simulink model "EulerPIDJoint_Tmp"  (Simulink 7.6)
settings: Solver=ode45  StartTime=0.0  StopTime=8  RelTol=1e-3
InitFcn:
  | eval('Config')
values from neighbouring files (symbols this model uses):
  a2 = 0    [Config.m]    (also in CtrPlatformCfg.m)
  a3 = 0    [Config.m]    (also in CtrPlatformCfg.m)
  a4 = 0    [Config.m]    (also in CtrPlatformCfg.m)
  a5 = 90    [Config.m]    (also in CtrPlatformCfg.m)
  a6 = 0    [Config.m]    (also in CtrPlatformCfg.m)
  Cen_EU = Cen    [DynEulerTest.m]
  DH_EU = [266     300     0       0       1016     0      174 ... (first row only)    [DynEulerTest.m]
  freq = tvel/radius    (= 1)    [Config.m]    (also in CtrPlatformCfg.m)
  Ft_EU = [0;0;0;0;0;0]    [DynEulerTest.m]
  Gravity = 9.8    [Config.m]    (also in CtrPlatformCfg.m)
  Ie_EU = [Ie1;Ie2;Ie3;Ie4;Ie5;Ie6]    [DynEulerTest.m]
  in1 = [5.2954 -0.2565 -0.6366;-0.2565 4.7000 0.2830;-0.6366 0.2829 5.8635]    [Config.m]    (also in CtrPlatformCfg.m; DynEulerTest.m; EfDynCAD.m = [0.54  -0.01 0.23)
  in2 = [5.8840 0.0072 0.0135;0.0072 6.0178 -0.1907;0.0135 -0.1907 0.3374]    [Config.m]    (also in CtrPlatformCfg.m; DynEulerTest.m; EfDynCAD.m = (R_x*R_z)*in2*(R_x*R_z)')
  in3 = [1.8201 -0.2274 -0.3112;-0.2274 2.2537 -0.1441;-0.3112 -0.1441 1.9485]    [Config.m]    (also in CtrPlatformCfg.m; DynEulerTest.m; EfDynCAD.m = (R_x*R_z)*in3*(R_x*R_z)')
  in4 = [0.0607 -0.0922 0;-0.0922 1.4493 0;0 0 1.4620]    [Config.m]    (also in CtrPlatformCfg.m; DynEulerTest.m = [0.0607 -0.0922 0;-0.0922 1.4493 0;0 0,1.4620]; EfDynCAD.m = (R_y*Rz)*in4*(R_y*Rz)')
  in5 = [0.0191 0.0032 0;0.0032 0.0228 0;0 0 0.0291]    [Config.m]    (also in CtrPlatformCfg.m; DynEulerTest.m; EfDynCAD.m = (R_x*R_y)*in5*(R_x*R_y)')
  in6 = [0.0012 0 0;0 0.0007 0;0 0 0.0007]    [Config.m]    (also in CtrPlatformCfg.m; DynEulerTest.m; EfDynCAD.m = (R_y*Rz)*in6*(R_y*Rz)')
  init_Endx = gd_init(1,4)    [Config.m]    (also in CtrPlatformCfg.m)
  init_Endy = gd_init(2,4)    [Config.m]    (also in CtrPlatformCfg.m)
  init_Endz = gd_init(3,4)    [Config.m]    (also in CtrPlatformCfg.m)
  init_Rot = gd_init(1:3,1:3)    [Config.m]    (also in CtrPlatformCfg.m)
  L = [l1 l2 l3 l4 l5 l6 l7 l8 l9]    [Config.m]    (also in CtrPlatformCfg.m)
  ma1 = 170.31    [Config.m]    (also in CtrPlatformCfg.m; DynEulerTest.m; EfDynCAD.m = 77.75)
  ma2 = 63.74    [Config.m]    (also in CtrPlatformCfg.m; DynEulerTest.m; EfDynCAD.m = 32.31)
  ma3 = 98.98    [Config.m]    (also in CtrPlatformCfg.m; DynEulerTest.m; EfDynCAD.m = 18.61)
  ma4 = 24.46    [Config.m]    (also in CtrPlatformCfg.m; DynEulerTest.m; EfDynCAD.m = 15.65)
  ma5 = 5.24    [Config.m]    (also in CtrPlatformCfg.m; DynEulerTest.m; EfDynCAD.m = 3.32)
  ma6 = 0.6    [Config.m]    (also in CtrPlatformCfg.m; DynEulerTest.m; EfDynCAD.m)
  Ma_EU = Ma    [DynEulerTest.m]
  tvel = 120    [Config.m]    (also in CtrPlatformCfg.m)
undefined symbols (not defined in the file or in its folder): a1
libraries: mblibv1 x41, simulink x4
(part 3 of 4)

== system EulerPIDJoint_Tmp/Display/GeneralVelDisplay/Jnt6 ==
  Enc : Inport
  Ref : Inport  Port=2
  Demux1 : Demux  Outputs=2
  Demux3 : Demux  Outputs=6
  Display : Subsystem
  Mux : Mux  Inputs=3
  Mux1 : Mux  Inputs=3
  Mux2 : Mux  Inputs=2
  Mux3 : Mux  Inputs=2
  Sign{1,3..4,6} (4 alike) : Gain
  Sign2 : Gain  Gain=-1
  Sign5 : Gain  Gain=-1
  wires:
  Mux3/1 -> Display/2(Ref_GeneralVel6)
  Mux2/1 -> Display/1(GeneralVel6)
  Sign5/1 -> Mux1/2
  Sign2/1 -> Mux/2
  Demux3/6 -> Sign6/1
  Demux3/5 -> Sign5/1
  Demux3/4 -> Sign4/1
  Demux3/3 -> Sign3/1
  Demux3/2 -> Sign2/1
  Demux3/1 -> Sign1/1
  Mux1/1 -> Mux3/2
  Mux/1 -> Mux3/1
  Ref/1 -> Demux3/1
  Enc/1 -> Demux1/1
  Sign1/1 -> Mux/3
  Sign3/1 -> Mux/1
  Sign6/1 -> Mux1/1
  Sign4/1 -> Mux1/3
  Demux1/1 -> Mux2/1
  Demux1/2 -> Mux2/2

== system EulerPIDJoint_Tmp/Display/JntVelAccDisplay/Joint1 ==
  JVA1 : Inport
  Ref_JVA1 : Inport  Port=2
  Acceleration : Scope  NumInputPorts=2
      settings: YMin=-5~-5  YMax=5~5  SaveName=ScopeData2
  Angle : Scope  NumInputPorts=2
      settings: TimeRange=10  YMin=-2.999999999999999e-017~-1  YMax=4e-017~1
  Demux : Demux  Outputs=3
  Demux1 : Demux  Outputs=3
  "Encoder " : ToWorkspace  VariableName=EncJVAJ1  SampleTime=-1  SaveFormat=Structure
  Err1 : Scope
      settings: SaveName=ScopeData6
  Err2 : Scope
      settings: SaveName=ScopeData7
  Err3 : Scope
      settings: SaveName=ScopeData8
  "Ref " : ToWorkspace  VariableName=RefJVAJ1  SampleTime=-1  SaveFormat=Structure
  Sum : Sum  Inputs=+|-
  Sum1 : Sum  Inputs=+|-
  Sum2 : Sum  Inputs=+|-
  "Velocity " : Scope  NumInputPorts=2
      settings: YMin=-5~-5  YMax=5~5
  wires:
  Ref_JVA1/1 -> "Ref "/1, Demux1/1
  JVA1/1 -> "Encoder "/1, Demux/1
  Sum2/1 -> Err3/1
  Sum1/1 -> Err2/1
  Sum/1 -> Err1/1
  Demux/1 -> Angle/1, Sum/1
  Demux1/1 -> Angle/2, Sum/2
  Demux/2 -> "Velocity "/1, Sum1/1
  Demux1/2 -> "Velocity "/2, Sum1/2
  Demux/3 -> Acceleration/1, Sum2/1
  Demux1/3 -> Acceleration/2, Sum2/2

== system EulerPIDJoint_Tmp/Display/JntVelAccDisplay/Joint2 ==
  JVA2 : Inport
  Ref_JVA2 : Inport  Port=2
  Acceleration : Scope  NumInputPorts=2
      settings: YMin=-5~-5  YMax=5~5  SaveName=ScopeData2
  Angle : Scope  NumInputPorts=2
      settings: TimeRange=10  YMin=-2.999999999999999e-017~-1  YMax=4e-017~1
  Demux : Demux  Outputs=3
  Demux1 : Demux  Outputs=3
  "Encoder " : ToWorkspace  VariableName=EncJVAJ2  SampleTime=-1  SaveFormat=Structure
  Err1 : Scope
      settings: SaveName=ScopeData6
  Err2 : Scope
      settings: SaveName=ScopeData7
  Err3 : Scope
      settings: SaveName=ScopeData8
  "Ref " : ToWorkspace  VariableName=RefJVAJ2  SampleTime=-1  SaveFormat=Structure
  Sum : Sum  Inputs=+|-
  Sum1 : Sum  Inputs=+|-
  Sum2 : Sum  Inputs=+|-
  "Velocity " : Scope  NumInputPorts=2
      settings: YMin=-5~-5  YMax=5~5
  wires:
  Demux1/3 -> Sum2/2, Acceleration/2
  Demux/3 -> Sum2/1, Acceleration/1
  Demux1/2 -> Sum1/2, "Velocity "/2
  Demux/2 -> Sum1/1, "Velocity "/1
  Demux1/1 -> Sum/2, Angle/2
  Demux/1 -> Sum/1, Angle/1
  Sum/1 -> Err1/1
  Sum1/1 -> Err2/1
  Sum2/1 -> Err3/1
  JVA2/1 -> Demux/1, "Encoder "/1
  Ref_JVA2/1 -> Demux1/1, "Ref "/1

== system EulerPIDJoint_Tmp/Display/JntVelAccDisplay/Joint3 ==
  JVA3 : Inport
  Ref_JVA3 : Inport  Port=2
  Acceleration : Scope  NumInputPorts=2
      settings: YMin=-5~-5  YMax=5~5  SaveName=ScopeData2
  Angle : Scope  NumInputPorts=2
      settings: TimeRange=10  YMin=-2.999999999999999e-017~-1  YMax=4e-017~1
  Demux : Demux  Outputs=3
  Demux1 : Demux  Outputs=3
  "Encoder " : ToWorkspace  VariableName=EncJVAJ3  SampleTime=-1  SaveFormat=Structure
  Err1 : Scope
      settings: SaveName=ScopeData6
  Err2 : Scope
      settings: SaveName=ScopeData7
  Err3 : Scope
      settings: SaveName=ScopeData8
  "Ref " : ToWorkspace  VariableName=RefJVAJ3  SampleTime=-1  SaveFormat=Structure
  Sum : Sum  Inputs=+|-
  Sum1 : Sum  Inputs=+|-
  Sum2 : Sum  Inputs=+|-
  "Velocity " : Scope  NumInputPorts=2
      settings: YMin=-5~-5  YMax=5~5
  wires:
  Ref_JVA3/1 -> "Ref "/1, Demux1/1
  JVA3/1 -> "Encoder "/1, Demux/1
  Sum2/1 -> Err3/1
  Sum1/1 -> Err2/1
  Sum/1 -> Err1/1
  Demux/1 -> Angle/1, Sum/1
  Demux1/1 -> Angle/2, Sum/2
  Demux/2 -> "Velocity "/1, Sum1/1
  Demux1/2 -> "Velocity "/2, Sum1/2
  Demux/3 -> Acceleration/1, Sum2/1
  Demux1/3 -> Acceleration/2, Sum2/2

== system EulerPIDJoint_Tmp/Display/JntVelAccDisplay/Joint4 ==
  JVA4 : Inport
  Ref_JVA4 : Inport  Port=2
  Acceleration : Scope  NumInputPorts=2
      settings: YMin=-5~-5  YMax=5~5  SaveName=ScopeData2
  Angle : Scope  NumInputPorts=2
      settings: TimeRange=10  YMin=-2.999999999999999e-017~-1  YMax=4e-017~1
  Demux : Demux  Outputs=3
  Demux1 : Demux  Outputs=3
  "Encoder " : ToWorkspace  VariableName=EncJVAJ4  SampleTime=-1  SaveFormat=Structure
  Err1 : Scope
      settings: SaveName=ScopeData6
  Err2 : Scope
      settings: SaveName=ScopeData7
  Err3 : Scope
      settings: SaveName=ScopeData8
  "Ref " : ToWorkspace  VariableName=RefJVAJ4  SampleTime=-1  SaveFormat=Structure
  Sum : Sum  Inputs=+|-
  Sum1 : Sum  Inputs=+|-
  Sum2 : Sum  Inputs=+|-
  "Velocity " : Scope  NumInputPorts=2
      settings: YMin=-5~-5  YMax=5~5
  wires:
  Demux1/3 -> Sum2/2, Acceleration/2
  Demux/3 -> Sum2/1, Acceleration/1
  Demux1/2 -> Sum1/2, "Velocity "/2
  Demux/2 -> Sum1/1, "Velocity "/1
  Demux1/1 -> Sum/2, Angle/2
  Demux/1 -> Sum/1, Angle/1
  Sum/1 -> Err1/1
  Sum1/1 -> Err2/1
  Sum2/1 -> Err3/1
  JVA4/1 -> Demux/1, "Encoder "/1
  Ref_JVA4/1 -> Demux1/1, "Ref "/1

== system EulerPIDJoint_Tmp/Display/JntVelAccDisplay/Joint5 ==
  JVA5 : Inport
  Ref_JVA5 : Inport  Port=2
  Acceleration : Scope  NumInputPorts=2
      settings: YMin=-5~-5  YMax=5~5  SaveName=ScopeData2
  Angle : Scope  NumInputPorts=2
      settings: TimeRange=10  YMin=-2.999999999999999e-017~-1  YMax=4e-017~1
  Demux : Demux  Outputs=3
  Demux1 : Demux  Outputs=3
  "Encoder " : ToWorkspace  VariableName=EncJVAJ5  SampleTime=-1  SaveFormat=Structure
  Err1 : Scope
      settings: SaveName=ScopeData6
  Err2 : Scope
      settings: SaveName=ScopeData7
  Err3 : Scope
      settings: SaveName=ScopeData8
  "Ref " : ToWorkspace  VariableName=RefJVAJ5  SampleTime=-1  SaveFormat=Structure
  Sum : Sum  Inputs=+|-
  Sum1 : Sum  Inputs=+|-
  Sum2 : Sum  Inputs=+|-
  "Velocity " : Scope  NumInputPorts=2
      settings: YMin=-5~-5  YMax=5~5
  wires:
  Ref_JVA5/1 -> "Ref "/1, Demux1/1
  JVA5/1 -> "Encoder "/1, Demux/1
  Sum2/1 -> Err3/1
  Sum1/1 -> Err2/1
  Sum/1 -> Err1/1
  Demux/1 -> Angle/1, Sum/1
  Demux1/1 -> Angle/2, Sum/2
  Demux/2 -> "Velocity "/1, Sum1/1
  Demux1/2 -> "Velocity "/2, Sum1/2
  Demux/3 -> Acceleration/1, Sum2/1
  Demux1/3 -> Acceleration/2, Sum2/2

== system EulerPIDJoint_Tmp/Display/JntVelAccDisplay/Joint6 ==
  JVA6 : Inport
  Ref_JVA6 : Inport  Port=2
  Acceleration : Scope  NumInputPorts=2
      settings: YMin=-5~-5  YMax=5~5  SaveName=ScopeData2
  Angle : Scope  NumInputPorts=2
      settings: TimeRange=10  YMin=-2.999999999999999e-017~-1  YMax=4e-017~1
  Demux : Demux  Outputs=3
  Demux1 : Demux  Outputs=3
  "Encoder " : ToWorkspace  VariableName=EncJVAJ6  SampleTime=-1  SaveFormat=Structure
  Err1 : Scope
      settings: SaveName=ScopeData6
  Err2 : Scope
      settings: SaveName=ScopeData7
  Err3 : Scope
      settings: SaveName=ScopeData8
  "Ref " : ToWorkspace  VariableName=RefJVAJ6  SampleTime=-1  SaveFormat=Structure
  Sum : Sum  Inputs=+|-
  Sum1 : Sum  Inputs=+|-
  Sum2 : Sum  Inputs=+|-
  "Velocity " : Scope  NumInputPorts=2
      settings: YMin=-5~-5  YMax=5~5
  wires:
  Demux1/3 -> Sum2/2, Acceleration/2
  Demux/3 -> Sum2/1, Acceleration/1
  Demux1/2 -> Sum1/2, "Velocity "/2
  Demux/2 -> Sum1/1, "Velocity "/1
  Demux1/1 -> Sum/2, Angle/2
  Demux/1 -> Sum/1, Angle/1
  Sum/1 -> Err1/1
  Sum1/1 -> Err2/1
  Sum2/1 -> Err3/1
  JVA6/1 -> Demux/1, "Encoder "/1
  Ref_JVA6/1 -> Demux1/1, "Ref "/1

== system EulerPIDJoint_Tmp/Trajectory Generator/Circle in Descartes Space/EndVelocity ==
  Constant : Constant  Value=-1
  End_Vx : Sin  Amplitude=-tvel  Frequency=freq  SampleTime=0
  End_Vy : Sin  Frequency=freq  Phase=pi/2  SampleTime=0
  End_Vz : Constant  Value=0
  Gain : Gain  Gain=tvel
  Ramp : simulink/Sources/Ramp  SystemSampleTime=-1  slope=1  start=0  X0=0
  Ramp1 : simulink/Sources/Ramp  SystemSampleTime=-1  slope=-1  start=1  X0=0
  Sum : Sum  Inputs=|++
  Sum1 : Sum  Inputs=++|
  Sum2 : Sum  Inputs=++|
  Transport Delay : TransportDelay
  Transport Delay1 : TransportDelay
  EndVx : Outport
  EndVy : Outport  Port=2
  EndVz : Outport  Port=3
  wires:
  End_Vy/1 -> Sum2/1
  Ramp/1 -> Sum/1
  Ramp1/1 -> Sum/2
  Transport Delay/1 -> Sum1/1
  Sum2/1 -> Transport Delay/1
  Constant/1 -> Sum2/2
  Sum/1 -> Sum1/2
  Sum1/1 -> Gain/1
  End_Vx/1 -> Transport Delay1/1
  Gain/1 -> EndVy/1
  End_Vz/1 -> EndVx/1
  Transport Delay1/1 -> EndVz/1

== system EulerPIDJoint_Tmp/Trajectory Generator/Circle in Descartes Space/Re-group  ==
  JJVVAA : Inport
  Demux2 : Demux  Outputs=18
  Mux{,1..2,4..6} (6 alike) : Mux  Inputs=3
  Mux3 : Mux  Inputs=6
  JVAJVA : Outport
  wires:
  JJVVAA/1 -> Demux2/1
  Mux3/1 -> JVAJVA/1
  Mux/1 -> Mux3/1
  Mux1/1 -> Mux3/2
  Mux2/1 -> Mux3/3
  Mux4/1 -> Mux3/4
  Mux5/1 -> Mux3/5
  Mux6/1 -> Mux3/6
  Demux2/1 -> Mux/1
  Demux2/2 -> Mux1/1
  Demux2/3 -> Mux2/1
  Demux2/4 -> Mux4/1
  Demux2/5 -> Mux5/1
  Demux2/6 -> Mux6/1
  Demux2/7 -> Mux/2
  Demux2/8 -> Mux1/2
  Demux2/9 -> Mux2/2
  Demux2/10 -> Mux4/2
  Demux2/11 -> Mux5/2
  Demux2/12 -> Mux6/2
  Demux2/13 -> Mux/3
  Demux2/14 -> Mux1/3
  Demux2/15 -> Mux2/3
  Demux2/16 -> Mux4/3
  Demux2/17 -> Mux5/3
  Demux2/18 -> Mux6/3

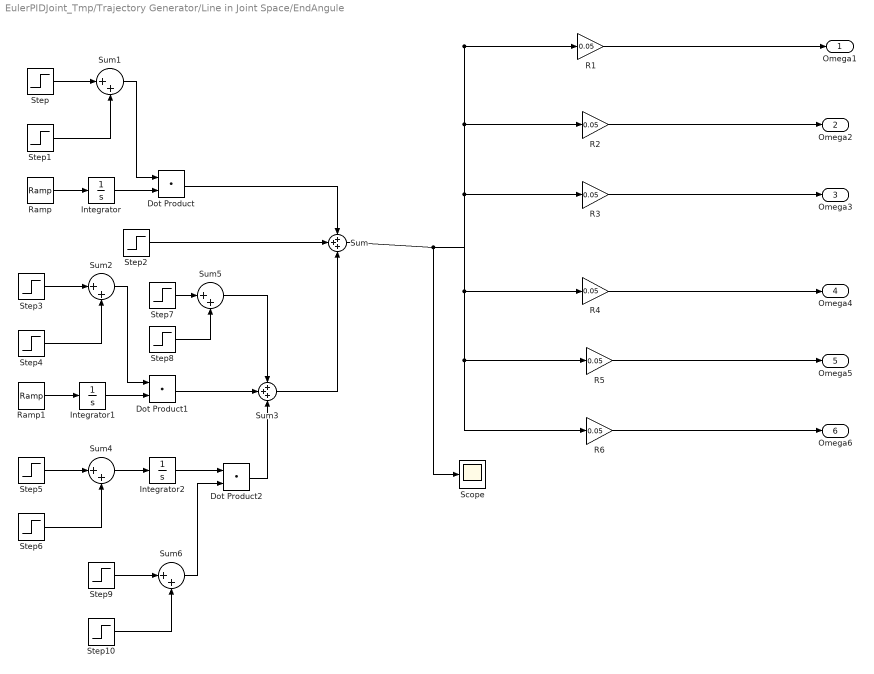
== system EulerPIDJoint_Tmp/Trajectory Generator/Line in Joint Space/EndAngule ==
  Dot Product : DotProduct  InputSameDT=on  OutDataTypeStr=Inherit: Inherit via internal rule
  Dot Product1 : DotProduct  InputSameDT=on  OutDataTypeStr=Inherit: Inherit via internal rule
  Dot Product2 : DotProduct  InputSameDT=on  OutDataTypeStr=Inherit: Inherit via internal rule
  Integrator : Integrator
  Integrator1 : Integrator
  Integrator2 : Integrator
  R{1..6} (6 alike) : Gain  Gain=0.05
  Ramp : simulink/Sources/Ramp  SystemSampleTime=-1  slope=1  start=0  X0=0
  Ramp1 : simulink/Sources/Ramp  SystemSampleTime=-1  slope=-1  start=0  X0=0
  Scope : Scope
      settings: SaveName=ScopeData21
  Step : Step  After=-1  SampleTime=0
  Step1 : Step  Time=0  SampleTime=0
  Step10 : Step  SampleTime=0
  Step2 : Step  Time=2  SampleTime=0
  Step3 : Step  Time=2  After=-1  SampleTime=0
  Step4 : Step  SampleTime=0
  Step5 : Step  Time=2  After=-2  SampleTime=0
  Step6 : Step  After=2  SampleTime=0
  Step7 : Step  Time=2  After=-1  SampleTime=0
  Step8 : Step  SampleTime=0
  Step9 : Step  Time=2  After=-1  SampleTime=0
  Sum : Sum  Inputs=+++
  Sum{1..2,4..6} (5 alike) : Sum  Inputs=|++
  Sum3 : Sum  Inputs=+++
  Omega1 : Outport
  Omega2 : Outport  Port=2
  Omega3 : Outport  Port=3
  Omega4 : Outport  Port=4
  Omega5 : Outport  Port=5
  Omega6 : Outport  Port=6
  wires:
  R4/1 -> Omega4/1
  R6/1 -> Omega6/1
  R5/1 -> Omega5/1
  R3/1 -> Omega3/1
  R2/1 -> Omega2/1
  Ramp/1 -> Integrator/1
  R1/1 -> Omega1/1
  Sum/1 -> R1/1, R2/1, R3/1, R4/1, R5/1, R6/1, Scope/1
  Integrator/1 -> Dot Product/2
  Step/1 -> Sum1/1
  Sum1/1 -> Dot Product/1
  Step1/1 -> Sum1/2
  Dot Product/1 -> Sum/1
  Step2/1 -> Sum/2
  Ramp1/1 -> Integrator1/1
  Integrator1/1 -> Dot Product1/2
  Step3/1 -> Sum2/1
  Sum2/1 -> Dot Product1/1
  Step4/1 -> Sum2/2
  Sum3/1 -> Sum/3
  Step5/1 -> Sum4/1
  Step6/1 -> Sum4/2
  Sum4/1 -> Integrator2/1
  Dot Product1/1 -> Sum3/2
  Step7/1 -> Sum5/1
  Step8/1 -> Sum5/2
  Sum5/1 -> Sum3/1
  Step9/1 -> Sum6/1
  Step10/1 -> Sum6/2
  Integrator2/1 -> Dot Product2/1
  Sum6/1 -> Dot Product2/2
  Dot Product2/1 -> Sum3/3

== system EulerPIDJoint_Tmp/Trajectory Generator/Line in Joint Space/Re-group  ==
  JJVVAA : Inport
  Demux2 : Demux  Outputs=18
  Mux{,1..2,4..6} (6 alike) : Mux  Inputs=3
  Mux3 : Mux  Inputs=6
  JVAJVA : Outport
  wires:
  JJVVAA/1 -> Demux2/1
  Mux3/1 -> JVAJVA/1
  Mux/1 -> Mux3/1
  Mux1/1 -> Mux3/2
  Mux2/1 -> Mux3/3
  Mux4/1 -> Mux3/4
  Mux5/1 -> Mux3/5
  Mux6/1 -> Mux3/6
  Demux2/1 -> Mux/1
  Demux2/2 -> Mux1/1
  Demux2/3 -> Mux2/1
  Demux2/4 -> Mux4/1
  Demux2/5 -> Mux5/1
  Demux2/6 -> Mux6/1
  Demux2/7 -> Mux/2
  Demux2/8 -> Mux1/2
  Demux2/9 -> Mux2/2
  Demux2/10 -> Mux4/2
  Demux2/11 -> Mux5/2
  Demux2/12 -> Mux6/2
  Demux2/13 -> Mux/3
  Demux2/14 -> Mux1/3
  Demux2/15 -> Mux2/3
  Demux2/16 -> Mux4/3
  Demux2/17 -> Mux5/3
  Demux2/18 -> Mux6/3

== system EulerPIDJoint_Tmp/Trajectory Generator/Sampled Trajectory Data/Re-group  ==
  JJVVAA : Inport
  Demux2 : Demux  Outputs=18
  Mux{,1..2,4..6} (6 alike) : Mux  Inputs=3
  Mux3 : Mux  Inputs=6
  JVAJVA : Outport
  wires:
  JJVVAA/1 -> Demux2/1
  Mux3/1 -> JVAJVA/1
  Mux/1 -> Mux3/1
  Mux1/1 -> Mux3/2
  Mux2/1 -> Mux3/3
  Mux4/1 -> Mux3/4
  Mux5/1 -> Mux3/5
  Mux6/1 -> Mux3/6
  Demux2/1 -> Mux/1
  Demux2/2 -> Mux1/1
  Demux2/3 -> Mux2/1
  Demux2/4 -> Mux4/1
  Demux2/5 -> Mux5/1
  Demux2/6 -> Mux6/1
  Demux2/7 -> Mux/2
  Demux2/8 -> Mux1/2
  Demux2/9 -> Mux2/2
  Demux2/10 -> Mux4/2
  Demux2/11 -> Mux5/2
  Demux2/12 -> Mux6/2
  Demux2/13 -> Mux/3
  Demux2/14 -> Mux1/3
  Demux2/15 -> Mux2/3
  Demux2/16 -> Mux4/3
  Demux2/17 -> Mux5/3
  Demux2/18 -> Mux6/3

== system EulerPIDJoint_Tmp/Trajectory Generator/Still/EndVelocity ==
  Constant : Constant  Value=0
  Constant1 : Constant  Value=0
  Constant2 : Constant  Value=0
  EndVx : Outport
  EndVy : Outport  Port=2
  EndVz : Outport  Port=3
  wires:
  Constant/1 -> EndVx/1
  Constant1/1 -> EndVy/1
  Constant2/1 -> EndVz/1

== system EulerPIDJoint_Tmp/Trajectory Generator/Still/Re-group  ==
  JJVVAA : Inport
  Demux2 : Demux  Outputs=18
  Mux{,1..2,4..6} (6 alike) : Mux  Inputs=3
  Mux3 : Mux  Inputs=6
  JVAJVA : Outport
  wires:
  Demux2/18 -> Mux6/3
  Demux2/17 -> Mux5/3
  Demux2/16 -> Mux4/3
  Demux2/15 -> Mux2/3
  Demux2/14 -> Mux1/3
  Demux2/13 -> Mux/3
  Demux2/12 -> Mux6/2
  Demux2/11 -> Mux5/2
  Demux2/10 -> Mux4/2
  Demux2/9 -> Mux2/2
  Demux2/8 -> Mux1/2
  Demux2/7 -> Mux/2
  Demux2/6 -> Mux6/1
  Demux2/5 -> Mux5/1
  Demux2/4 -> Mux4/1
  Demux2/3 -> Mux2/1
  Demux2/2 -> Mux1/1
  Demux2/1 -> Mux/1
  Mux6/1 -> Mux3/6
  Mux5/1 -> Mux3/5
  Mux4/1 -> Mux3/4
  Mux2/1 -> Mux3/3
  Mux1/1 -> Mux3/2
  Mux/1 -> Mux3/1
  Mux3/1 -> JVAJVA/1
  JJVVAA/1 -> Demux2/1

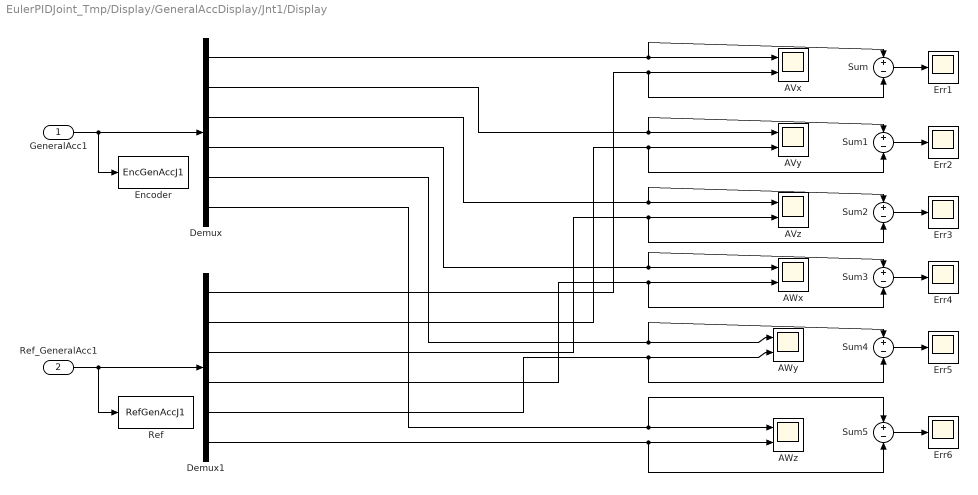
== system EulerPIDJoint_Tmp/Display/GeneralAccDisplay/Jnt1/Display ==
  GeneralAcc1 : Inport
  Ref_GeneralAcc1 : Inport  Port=2
  AVx : Scope  NumInputPorts=2
      settings: TimeRange=10  YMin=-2.999999999999999e-017~-1  YMax=4e-017~1
  "AVy " : Scope  NumInputPorts=2
      settings: YMin=-5~-5  YMax=5~5
  AVz : Scope  NumInputPorts=2
      settings: YMin=-5~-5  YMax=5~5  SaveName=ScopeData2
  AWx : Scope  NumInputPorts=2
      settings: YMin=-5~-5  YMax=5~5  SaveName=ScopeData3
  AWy : Scope  NumInputPorts=2
      settings: TimeRange=10  YMin=-4.18~4.060000000000001  YMax=-4.04~4.2  SaveName=ScopeData4
  AWz : Scope  NumInputPorts=2
      settings: TimeRange=10  YMin=-1.6e-006~-0.003  YMax=4e-007~0.004  SaveName=ScopeData5
  Demux : Demux  Outputs=6
  Demux1 : Demux  Outputs=6
  "Encoder " : ToWorkspace  VariableName=EncGenAccJ1  SampleTime=-1  SaveFormat=Structure
  Err{1..6} (6 alike) : Scope
      Err1 settings: SaveName=ScopeData6
      Err2 settings: SaveName=ScopeData7
      Err3 settings: SaveName=ScopeData8
      Err4 settings: SaveName=ScopeData9
      Err5 settings: TimeRange=3  YMin=-2.5  YMax=1  SaveName=ScopeData10
      Err6 settings: SaveName=ScopeData11
  "Ref " : ToWorkspace  VariableName=RefGenAccJ1  SampleTime=-1  SaveFormat=Structure
  Sum{,1..5} (6 alike) : Sum  Inputs=+|-
  wires:
  Demux1/6 -> Sum5/2, AWz/2
  Demux1/5 -> Sum4/2, AWy/2
  Demux1/4 -> AWx/2, Sum3/2
  Demux1/3 -> Sum2/2, AVz/2
  Demux1/2 -> Sum1/2, "AVy "/2
  Demux/6 -> Sum5/1, AWz/1
  Demux/5 -> Sum4/1, AWy/1
  Demux/4 -> AWx/1, Sum3/1
  Demux/3 -> Sum2/1, AVz/1
  Demux/2 -> Sum1/1, "AVy "/1
  Demux1/1 -> AVx/2, Sum/2
  Demux/1 -> AVx/1, Sum/1
  Ref_GeneralAcc1/1 -> "Ref "/1, Demux1/1
  GeneralAcc1/1 -> "Encoder "/1, Demux/1
  Sum5/1 -> Err6/1
  Sum4/1 -> Err5/1
  Sum3/1 -> Err4/1
  Sum2/1 -> Err3/1
  Sum1/1 -> Err2/1
  Sum/1 -> Err1/1

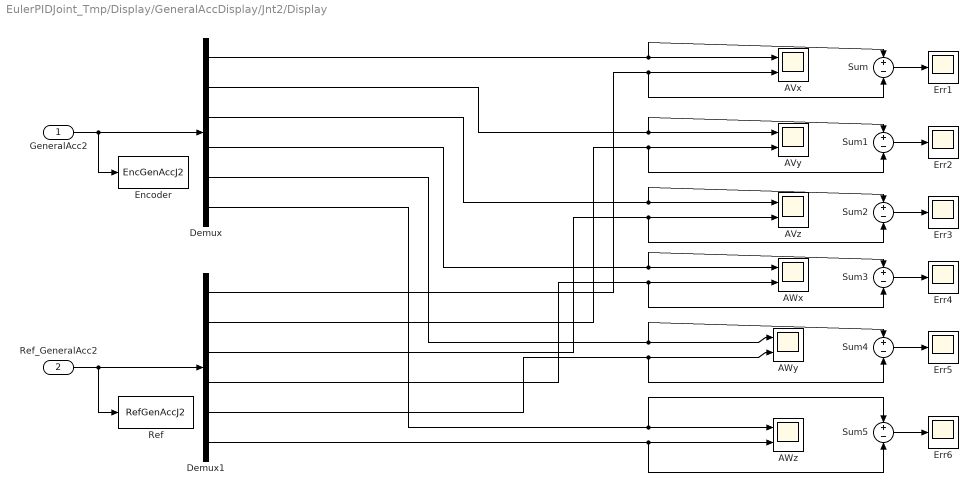
== system EulerPIDJoint_Tmp/Display/GeneralAccDisplay/Jnt2/Display ==
  GeneralAcc2 : Inport
  Ref_GeneralAcc2 : Inport  Port=2
  AVx : Scope  NumInputPorts=2
      settings: TimeRange=10  YMin=-2.999999999999999e-017~-1  YMax=4e-017~1
  "AVy " : Scope  NumInputPorts=2
      settings: YMin=-5~-5  YMax=5~5
  AVz : Scope  NumInputPorts=2
      settings: YMin=-5~-5  YMax=5~5  SaveName=ScopeData2
  AWx : Scope  NumInputPorts=2
      settings: YMin=-5~-5  YMax=5~5  SaveName=ScopeData3
  AWy : Scope  NumInputPorts=2
      settings: TimeRange=10  YMin=-4.18~4.060000000000001  YMax=-4.04~4.2  SaveName=ScopeData4
  AWz : Scope  NumInputPorts=2
      settings: TimeRange=10  YMin=-1.6e-006~-0.003  YMax=4e-007~0.004  SaveName=ScopeData5
  Demux : Demux  Outputs=6
  Demux1 : Demux  Outputs=6
  "Encoder " : ToWorkspace  VariableName=EncGenAccJ2  SampleTime=-1  SaveFormat=Structure
  Err{1..6} (6 alike) : Scope
      Err1 settings: SaveName=ScopeData6
      Err2 settings: SaveName=ScopeData7
      Err3 settings: SaveName=ScopeData8
      Err4 settings: SaveName=ScopeData9
      Err5 settings: TimeRange=3  YMin=-2.5  YMax=1  SaveName=ScopeData10
      Err6 settings: SaveName=ScopeData11
  "Ref " : ToWorkspace  VariableName=RefGenAccJ2  SampleTime=-1  SaveFormat=Structure
  Sum{,1..5} (6 alike) : Sum  Inputs=+|-
  wires:
  Sum/1 -> Err1/1
  Sum1/1 -> Err2/1
  Sum2/1 -> Err3/1
  Sum3/1 -> Err4/1
  Sum4/1 -> Err5/1
  Sum5/1 -> Err6/1
  GeneralAcc2/1 -> Demux/1, "Encoder "/1
  Ref_GeneralAcc2/1 -> Demux1/1, "Ref "/1
  Demux/1 -> Sum/1, AVx/1
  Demux1/1 -> Sum/2, AVx/2
  Demux/2 -> "AVy "/1, Sum1/1
  Demux/3 -> AVz/1, Sum2/1
  Demux/4 -> Sum3/1, AWx/1
  Demux/5 -> AWy/1, Sum4/1
  Demux/6 -> AWz/1, Sum5/1
  Demux1/2 -> "AVy "/2, Sum1/2
  Demux1/3 -> AVz/2, Sum2/2
  Demux1/4 -> Sum3/2, AWx/2
  Demux1/5 -> AWy/2, Sum4/2
  Demux1/6 -> AWz/2, Sum5/2

== system EulerPIDJoint_Tmp/Display/GeneralAccDisplay/Jnt3/Display ==
  GeneralAcc3 : Inport
  Ref_GeneralAcc3 : Inport  Port=2
  AVx : Scope  NumInputPorts=2
      settings: TimeRange=10  YMin=-2.999999999999999e-017~-1  YMax=4e-017~1
  "AVy " : Scope  NumInputPorts=2
      settings: YMin=-5~-5  YMax=5~5
  AVz : Scope  NumInputPorts=2
      settings: YMin=-5~-5  YMax=5~5  SaveName=ScopeData2
  AWx : Scope  NumInputPorts=2
      settings: YMin=-5~-5  YMax=5~5  SaveName=ScopeData3
  AWy : Scope  NumInputPorts=2
      settings: TimeRange=10  YMin=-4.18~4.060000000000001  YMax=-4.04~4.2  SaveName=ScopeData4
  AWz : Scope  NumInputPorts=2
      settings: TimeRange=10  YMin=-1.6e-006~-0.003  YMax=4e-007~0.004  SaveName=ScopeData5
  Demux : Demux  Outputs=6
  Demux1 : Demux  Outputs=6
  "Encoder " : ToWorkspace  VariableName=EncGenAccJ3  SampleTime=-1  SaveFormat=Structure
  Err{1..6} (6 alike) : Scope
      Err1 settings: SaveName=ScopeData6
      Err2 settings: SaveName=ScopeData7
      Err3 settings: SaveName=ScopeData8
      Err4 settings: SaveName=ScopeData9
      Err5 settings: TimeRange=3  YMin=-2.5  YMax=1  SaveName=ScopeData10
      Err6 settings: SaveName=ScopeData11
  "Ref " : ToWorkspace  VariableName=RefGenAccJ3  SampleTime=-1  SaveFormat=Structure
  Sum{,1..5} (6 alike) : Sum  Inputs=+|-
  wires:
  Demux1/6 -> Sum5/2, AWz/2
  Demux1/5 -> Sum4/2, AWy/2
  Demux1/4 -> AWx/2, Sum3/2
  Demux1/3 -> Sum2/2, AVz/2
  Demux1/2 -> Sum1/2, "AVy "/2
  Demux/6 -> Sum5/1, AWz/1
  Demux/5 -> Sum4/1, AWy/1
  Demux/4 -> AWx/1, Sum3/1
  Demux/3 -> Sum2/1, AVz/1
  Demux/2 -> Sum1/1, "AVy "/1
  Demux1/1 -> AVx/2, Sum/2
  Demux/1 -> AVx/1, Sum/1
  Ref_GeneralAcc3/1 -> "Ref "/1, Demux1/1
  GeneralAcc3/1 -> "Encoder "/1, Demux/1
  Sum5/1 -> Err6/1
  Sum4/1 -> Err5/1
  Sum3/1 -> Err4/1
  Sum2/1 -> Err3/1
  Sum1/1 -> Err2/1
  Sum/1 -> Err1/1

== system EulerPIDJoint_Tmp/Display/GeneralAccDisplay/Jnt4/Display ==
  GeneralAcc4 : Inport
  Ref_GeneralAcc4 : Inport  Port=2
  AVx : Scope  NumInputPorts=2
      settings: TimeRange=10  YMin=-2.999999999999999e-017~-1  YMax=4e-017~1
  "AVy " : Scope  NumInputPorts=2
      settings: YMin=-5~-5  YMax=5~5
  AVz : Scope  NumInputPorts=2
      settings: YMin=-5~-5  YMax=5~5  SaveName=ScopeData2
  AWx : Scope  NumInputPorts=2
      settings: YMin=-5~-5  YMax=5~5  SaveName=ScopeData3
  AWy : Scope  NumInputPorts=2
      settings: TimeRange=10  YMin=-4.18~4.060000000000001  YMax=-4.04~4.2  SaveName=ScopeData4
  AWz : Scope  NumInputPorts=2
      settings: TimeRange=10  YMin=-1.6e-006~-0.003  YMax=4e-007~0.004  SaveName=ScopeData5
  Demux : Demux  Outputs=6
  Demux1 : Demux  Outputs=6
  "Encoder " : ToWorkspace  VariableName=EncGenAccJ4  SampleTime=-1  SaveFormat=Structure
  Err{1..6} (6 alike) : Scope
      Err1 settings: SaveName=ScopeData6
      Err2 settings: SaveName=ScopeData7
      Err3 settings: SaveName=ScopeData8
      Err4 settings: SaveName=ScopeData9
      Err5 settings: TimeRange=3  YMin=-2.5  YMax=1  SaveName=ScopeData10
      Err6 settings: SaveName=ScopeData11
  "Ref " : ToWorkspace  VariableName=RefGenAccJ4  SampleTime=-1  SaveFormat=Structure
  Sum{,1..5} (6 alike) : Sum  Inputs=+|-
  wires:
  Sum/1 -> Err1/1
  Sum1/1 -> Err2/1
  Sum2/1 -> Err3/1
  Sum3/1 -> Err4/1
  Sum4/1 -> Err5/1
  Sum5/1 -> Err6/1
  GeneralAcc4/1 -> Demux/1, "Encoder "/1
  Ref_GeneralAcc4/1 -> Demux1/1, "Ref "/1
  Demux/1 -> Sum/1, AVx/1
  Demux1/1 -> Sum/2, AVx/2
  Demux/2 -> "AVy "/1, Sum1/1
  Demux/3 -> AVz/1, Sum2/1
  Demux/4 -> Sum3/1, AWx/1
  Demux/5 -> AWy/1, Sum4/1
  Demux/6 -> AWz/1, Sum5/1
  Demux1/2 -> "AVy "/2, Sum1/2
  Demux1/3 -> AVz/2, Sum2/2
  Demux1/4 -> Sum3/2, AWx/2
  Demux1/5 -> AWy/2, Sum4/2
  Demux1/6 -> AWz/2, Sum5/2

== system EulerPIDJoint_Tmp/Display/GeneralAccDisplay/Jnt5/Display ==
  GeneralAcc5 : Inport
  Ref_GeneralAcc5 : Inport  Port=2
  AVx : Scope  NumInputPorts=2
      settings: TimeRange=10  YMin=-2.999999999999999e-017~-1  YMax=4e-017~1
  "AVy " : Scope  NumInputPorts=2
      settings: YMin=-5~-5  YMax=5~5
  AVz : Scope  NumInputPorts=2
      settings: YMin=-5~-5  YMax=5~5  SaveName=ScopeData2
  AWx : Scope  NumInputPorts=2
      settings: YMin=-5~-5  YMax=5~5  SaveName=ScopeData3
  AWy : Scope  NumInputPorts=2
      settings: TimeRange=10  YMin=-4.18~4.060000000000001  YMax=-4.04~4.2  SaveName=ScopeData4
  AWz : Scope  NumInputPorts=2
      settings: TimeRange=10  YMin=-1.6e-006~-0.003  YMax=4e-007~0.004  SaveName=ScopeData5
  Demux : Demux  Outputs=6
  Demux1 : Demux  Outputs=6
  "Encoder " : ToWorkspace  VariableName=EncGenAccJ5  SampleTime=-1  SaveFormat=Structure
  Err{1..6} (6 alike) : Scope
      Err1 settings: SaveName=ScopeData6
      Err2 settings: SaveName=ScopeData7
      Err3 settings: SaveName=ScopeData8
      Err4 settings: SaveName=ScopeData9
      Err5 settings: TimeRange=3  YMin=-2.5  YMax=1  SaveName=ScopeData10
      Err6 settings: SaveName=ScopeData11
  "Ref " : ToWorkspace  VariableName=RefGenAccJ5  SampleTime=-1  SaveFormat=Structure
  Sum{,1..5} (6 alike) : Sum  Inputs=+|-
  wires:
  Demux1/6 -> Sum5/2, AWz/2
  Demux1/5 -> Sum4/2, AWy/2
  Demux1/4 -> AWx/2, Sum3/2
  Demux1/3 -> Sum2/2, AVz/2
  Demux1/2 -> Sum1/2, "AVy "/2
  Demux/6 -> Sum5/1, AWz/1
  Demux/5 -> Sum4/1, AWy/1
  Demux/4 -> AWx/1, Sum3/1
  Demux/3 -> Sum2/1, AVz/1
  Demux/2 -> Sum1/1, "AVy "/1
  Demux1/1 -> AVx/2, Sum/2
  Demux/1 -> AVx/1, Sum/1
  Ref_GeneralAcc5/1 -> "Ref "/1, Demux1/1
  GeneralAcc5/1 -> "Encoder "/1, Demux/1
  Sum5/1 -> Err6/1
  Sum4/1 -> Err5/1
  Sum3/1 -> Err4/1
  Sum2/1 -> Err3/1
  Sum1/1 -> Err2/1
  Sum/1 -> Err1/1

== system EulerPIDJoint_Tmp/Display/GeneralAccDisplay/Jnt6/Display ==
  GeneralAcc6 : Inport
  Ref_GeneralAcc6 : Inport  Port=2
  AVx : Scope  NumInputPorts=2
      settings: TimeRange=10  YMin=-2.999999999999999e-017~-1  YMax=4e-017~1
  "AVy " : Scope  NumInputPorts=2
      settings: YMin=-5~-5  YMax=5~5
  AVz : Scope  NumInputPorts=2
      settings: YMin=-5~-5  YMax=5~5  SaveName=ScopeData2
  AWx : Scope  NumInputPorts=2
      settings: YMin=-5~-5  YMax=5~5  SaveName=ScopeData3
  AWy : Scope  NumInputPorts=2
      settings: TimeRange=10  YMin=-4.18~4.060000000000001  YMax=-4.04~4.2  SaveName=ScopeData4
  AWz : Scope  NumInputPorts=2
      settings: TimeRange=10  YMin=-1.6e-006~-0.003  YMax=4e-007~0.004  SaveName=ScopeData5
  Demux : Demux  Outputs=6
  Demux1 : Demux  Outputs=6
  "Encoder " : ToWorkspace  VariableName=EncGenAccJ6  SampleTime=-1  SaveFormat=Structure
  Err{1..6} (6 alike) : Scope
      Err1 settings: SaveName=ScopeData6
      Err2 settings: SaveName=ScopeData7
      Err3 settings: SaveName=ScopeData8
      Err4 settings: SaveName=ScopeData9
      Err5 settings: TimeRange=3  YMin=-2.5  YMax=1  SaveName=ScopeData10
      Err6 settings: SaveName=ScopeData11
  "Ref " : ToWorkspace  VariableName=RefGenAccJ6  SampleTime=-1  SaveFormat=Structure
  Sum{,1..5} (6 alike) : Sum  Inputs=+|-
  wires:
  Sum/1 -> Err1/1
  Sum1/1 -> Err2/1
  Sum2/1 -> Err3/1
  Sum3/1 -> Err4/1
  Sum4/1 -> Err5/1
  Sum5/1 -> Err6/1
  GeneralAcc6/1 -> Demux/1, "Encoder "/1
  Ref_GeneralAcc6/1 -> Demux1/1, "Ref "/1
  Demux/1 -> Sum/1, AVx/1
  Demux1/1 -> Sum/2, AVx/2
  Demux/2 -> "AVy "/1, Sum1/1
  Demux/3 -> AVz/1, Sum2/1
  Demux/4 -> Sum3/1, AWx/1
  Demux/5 -> AWy/1, Sum4/1
  Demux/6 -> AWz/1, Sum5/1
  Demux1/2 -> "AVy "/2, Sum1/2
  Demux1/3 -> AVz/2, Sum2/2
  Demux1/4 -> Sum3/2, AWx/2
  Demux1/5 -> AWy/2, Sum4/2
  Demux1/6 -> AWz/2, Sum5/2

== system EulerPIDJoint_Tmp/Display/GeneralForceDisplay/Jnt1/Display ==
  GeneralForce1 : Inport
  Ref_GeneralForce1 : Inport  Port=2
  Demux : Demux  Outputs=6
  Demux1 : Demux  Outputs=6
  "Encoder " : ToWorkspace  VariableName=EncGenForceJ1  SampleTime=-1  SaveFormat=Structure
  Err{1..6} (6 alike) : Scope
      Err1 settings: SaveName=ScopeData6
      Err2 settings: SaveName=ScopeData7
      Err3 settings: SaveName=ScopeData8
      Err4 settings: SaveName=ScopeData9
      Err5 settings: TimeRange=3  YMin=-2.5  YMax=1  SaveName=ScopeData10
      Err6 settings: SaveName=ScopeData11
  "Ref " : ToWorkspace  VariableName=RefGenForceJ1  SampleTime=-1  SaveFormat=Structure
  Sum{,1..5} (6 alike) : Sum  Inputs=+|-
  fx : Scope  NumInputPorts=2
      settings: TimeRange=10  YMin=-2.999999999999999e-017~-1  YMax=4e-017~1
  "fy " : Scope  NumInputPorts=2
      settings: YMin=-5~-5  YMax=5~5
  fz : Scope  NumInputPorts=2
      settings: YMin=-5~-5  YMax=5~5  SaveName=ScopeData2
  taux : Scope  NumInputPorts=2
      settings: YMin=-5~-5  YMax=5~5  SaveName=ScopeData3
  tauy : Scope  NumInputPorts=2
      settings: TimeRange=10  YMin=-4.18~4.060000000000001  YMax=-4.04~4.2  SaveName=ScopeData4
  tauz : Scope  NumInputPorts=2
      settings: TimeRange=10  YMin=-1.6e-006~-0.003  YMax=4e-007~0.004  SaveName=ScopeData5
  wires:
  Sum/1 -> Err1/1
  Sum1/1 -> Err2/1
  Sum2/1 -> Err3/1
  Sum3/1 -> Err4/1
  Sum4/1 -> Err5/1
  Sum5/1 -> Err6/1
  GeneralForce1/1 -> Demux/1, "Encoder "/1
  Ref_GeneralForce1/1 -> Demux1/1, "Ref "/1
  Demux/1 -> Sum/1, fx/1
  Demux1/1 -> Sum/2, fx/2
  Demux/2 -> "fy "/1, Sum1/1
  Demux/3 -> fz/1, Sum2/1
  Demux/4 -> Sum3/1, taux/1
  Demux/5 -> tauy/1, Sum4/1
  Demux/6 -> tauz/1, Sum5/1
  Demux1/2 -> "fy "/2, Sum1/2
  Demux1/3 -> fz/2, Sum2/2
  Demux1/4 -> Sum3/2, taux/2
  Demux1/5 -> tauy/2, Sum4/2
  Demux1/6 -> tauz/2, Sum5/2

== system EulerPIDJoint_Tmp/Display/GeneralForceDisplay/Jnt2/Display ==
  GeneralForce2 : Inport
  Ref_GeneralForce2 : Inport  Port=2
  Demux : Demux  Outputs=6
  Demux1 : Demux  Outputs=6
  "Encoder " : ToWorkspace  VariableName=EncGenForceJ2  SampleTime=-1  SaveFormat=Structure
  Err{1..6} (6 alike) : Scope
      Err1 settings: SaveName=ScopeData6
      Err2 settings: SaveName=ScopeData7
      Err3 settings: SaveName=ScopeData8
      Err4 settings: SaveName=ScopeData9
      Err5 settings: TimeRange=3  YMin=-2.5  YMax=1  SaveName=ScopeData10
      Err6 settings: SaveName=ScopeData11
  "Ref " : ToWorkspace  VariableName=RefGenForceJ2  SampleTime=-1  SaveFormat=Structure
  Sum{,1..5} (6 alike) : Sum  Inputs=+|-
  fx : Scope  NumInputPorts=2
      settings: TimeRange=10  YMin=-2.999999999999999e-017~-1  YMax=4e-017~1
  "fy " : Scope  NumInputPorts=2
      settings: YMin=-5~-5  YMax=5~5
  fz : Scope  NumInputPorts=2
      settings: YMin=-5~-5  YMax=5~5  SaveName=ScopeData2
  taux : Scope  NumInputPorts=2
      settings: YMin=-5~-5  YMax=5~5  SaveName=ScopeData3
  tauy : Scope  NumInputPorts=2
      settings: TimeRange=10  YMin=-4.18~4.060000000000001  YMax=-4.04~4.2  SaveName=ScopeData4
  tauz : Scope  NumInputPorts=2
      settings: TimeRange=10  YMin=-1.6e-006~-0.003  YMax=4e-007~0.004  SaveName=ScopeData5
  wires:
  Sum/1 -> Err1/1
  Sum1/1 -> Err2/1
  Sum2/1 -> Err3/1
  Sum3/1 -> Err4/1
  Sum4/1 -> Err5/1
  Sum5/1 -> Err6/1
  GeneralForce2/1 -> Demux/1, "Encoder "/1
  Ref_GeneralForce2/1 -> Demux1/1, "Ref "/1
  Demux/1 -> Sum/1, fx/1
  Demux1/1 -> Sum/2, fx/2
  Demux/2 -> "fy "/1, Sum1/1
  Demux/3 -> fz/1, Sum2/1
  Demux/4 -> Sum3/1, taux/1
  Demux/5 -> tauy/1, Sum4/1
  Demux/6 -> tauz/1, Sum5/1
  Demux1/2 -> "fy "/2, Sum1/2
  Demux1/3 -> fz/2, Sum2/2
  Demux1/4 -> Sum3/2, taux/2
  Demux1/5 -> tauy/2, Sum4/2
  Demux1/6 -> tauz/2, Sum5/2

== system EulerPIDJoint_Tmp/Display/GeneralForceDisplay/Jnt3/Display ==
  GeneralForce3 : Inport
  Ref_GeneralForce3 : Inport  Port=2
  Demux : Demux  Outputs=6
  Demux1 : Demux  Outputs=6
  "Encoder " : ToWorkspace  VariableName=EncGenForceJ3  SampleTime=-1  SaveFormat=Structure
  Err{1..6} (6 alike) : Scope
      Err1 settings: SaveName=ScopeData6
      Err2 settings: SaveName=ScopeData7
      Err3 settings: SaveName=ScopeData8
      Err4 settings: SaveName=ScopeData9
      Err5 settings: TimeRange=3  YMin=-2.5  YMax=1  SaveName=ScopeData10
      Err6 settings: SaveName=ScopeData11
  "Ref " : ToWorkspace  VariableName=RefGenForceJ3  SampleTime=-1  SaveFormat=Structure
  Sum{,1..5} (6 alike) : Sum  Inputs=+|-
  fx : Scope  NumInputPorts=2
      settings: TimeRange=10  YMin=-2.999999999999999e-017~-1  YMax=4e-017~1
  "fy " : Scope  NumInputPorts=2
      settings: YMin=-5~-5  YMax=5~5
  fz : Scope  NumInputPorts=2
      settings: YMin=-5~-5  YMax=5~5  SaveName=ScopeData2
  taux : Scope  NumInputPorts=2
      settings: YMin=-5~-5  YMax=5~5  SaveName=ScopeData3
  tauy : Scope  NumInputPorts=2
      settings: TimeRange=10  YMin=-4.18~4.060000000000001  YMax=-4.04~4.2  SaveName=ScopeData4
  tauz : Scope  NumInputPorts=2
      settings: TimeRange=10  YMin=-1.6e-006~-0.003  YMax=4e-007~0.004  SaveName=ScopeData5
  wires:
  Sum/1 -> Err1/1
  Sum1/1 -> Err2/1
  Sum2/1 -> Err3/1
  Sum3/1 -> Err4/1
  Sum4/1 -> Err5/1
  Sum5/1 -> Err6/1
  GeneralForce3/1 -> Demux/1, "Encoder "/1
  Ref_GeneralForce3/1 -> Demux1/1, "Ref "/1
  Demux/1 -> Sum/1, fx/1
  Demux1/1 -> Sum/2, fx/2
  Demux/2 -> "fy "/1, Sum1/1
  Demux/3 -> fz/1, Sum2/1
  Demux/4 -> Sum3/1, taux/1
  Demux/5 -> tauy/1, Sum4/1
  Demux/6 -> tauz/1, Sum5/1
  Demux1/2 -> "fy "/2, Sum1/2
  Demux1/3 -> fz/2, Sum2/2
  Demux1/4 -> Sum3/2, taux/2
  Demux1/5 -> tauy/2, Sum4/2
  Demux1/6 -> tauz/2, Sum5/2

== system EulerPIDJoint_Tmp/Display/GeneralForceDisplay/Jnt4/Display ==
  GeneralForce4 : Inport
  Ref_GeneralForce4 : Inport  Port=2
  Demux : Demux  Outputs=6
  Demux1 : Demux  Outputs=6
  "Encoder " : ToWorkspace  VariableName=EncGenForceJ4  SampleTime=-1  SaveFormat=Structure
  Err{1..6} (6 alike) : Scope
      Err1 settings: SaveName=ScopeData6
      Err2 settings: SaveName=ScopeData7
      Err3 settings: SaveName=ScopeData8
      Err4 settings: SaveName=ScopeData9
      Err5 settings: TimeRange=3  YMin=-2.5  YMax=1  SaveName=ScopeData10
      Err6 settings: SaveName=ScopeData11
  "Ref " : ToWorkspace  VariableName=RefGenForceJ4  SampleTime=-1  SaveFormat=Structure
  Sum{,1..5} (6 alike) : Sum  Inputs=+|-
  fx : Scope  NumInputPorts=2
      settings: TimeRange=10  YMin=-2.999999999999999e-017~-1  YMax=4e-017~1
  "fy " : Scope  NumInputPorts=2
      settings: YMin=-5~-5  YMax=5~5
  fz : Scope  NumInputPorts=2
      settings: YMin=-5~-5  YMax=5~5  SaveName=ScopeData2
  taux : Scope  NumInputPorts=2
      settings: YMin=-5~-5  YMax=5~5  SaveName=ScopeData3
  tauy : Scope  NumInputPorts=2
      settings: TimeRange=10  YMin=-4.18~4.060000000000001  YMax=-4.04~4.2  SaveName=ScopeData4
  tauz : Scope  NumInputPorts=2
      settings: TimeRange=10  YMin=-1.6e-006~-0.003  YMax=4e-007~0.004  SaveName=ScopeData5
  wires:
  Sum/1 -> Err1/1
  Sum1/1 -> Err2/1
  Sum2/1 -> Err3/1
  Sum3/1 -> Err4/1
  Sum4/1 -> Err5/1
  Sum5/1 -> Err6/1
  GeneralForce4/1 -> Demux/1, "Encoder "/1
  Ref_GeneralForce4/1 -> Demux1/1, "Ref "/1
  Demux/1 -> Sum/1, fx/1
  Demux1/1 -> Sum/2, fx/2
  Demux/2 -> "fy "/1, Sum1/1
  Demux/3 -> fz/1, Sum2/1
  Demux/4 -> Sum3/1, taux/1
  Demux/5 -> tauy/1, Sum4/1
  Demux/6 -> tauz/1, Sum5/1
  Demux1/2 -> "fy "/2, Sum1/2
  Demux1/3 -> fz/2, Sum2/2
  Demux1/4 -> Sum3/2, taux/2
  Demux1/5 -> tauy/2, Sum4/2
  Demux1/6 -> tauz/2, Sum5/2

== system EulerPIDJoint_Tmp/Display/GeneralForceDisplay/Jnt5/Display ==
  GeneralForce5 : Inport
  Ref_GeneralForce5 : Inport  Port=2
  Demux : Demux  Outputs=6
  Demux1 : Demux  Outputs=6
  "Encoder " : ToWorkspace  VariableName=EncGenForceJ5  SampleTime=-1  SaveFormat=Structure
  Err{1..6} (6 alike) : Scope
      Err1 settings: SaveName=ScopeData6
      Err2 settings: SaveName=ScopeData7
      Err3 settings: SaveName=ScopeData8
      Err4 settings: SaveName=ScopeData9
      Err5 settings: TimeRange=3  YMin=-2.5  YMax=1  SaveName=ScopeData10
      Err6 settings: SaveName=ScopeData11
  "Ref " : ToWorkspace  VariableName=RefGenForceJ5  SampleTime=-1  SaveFormat=Structure
  Sum{,1..5} (6 alike) : Sum  Inputs=+|-
  fx : Scope  NumInputPorts=2
      settings: TimeRange=10  YMin=-2.999999999999999e-017~-1  YMax=4e-017~1
  "fy " : Scope  NumInputPorts=2
      settings: YMin=-5~-5  YMax=5~5
  fz : Scope  NumInputPorts=2
      settings: YMin=-5~-5  YMax=5~5  SaveName=ScopeData2
  taux : Scope  NumInputPorts=2
      settings: YMin=-5~-5  YMax=5~5  SaveName=ScopeData3
  tauy : Scope  NumInputPorts=2
      settings: TimeRange=10  YMin=-4.18~4.060000000000001  YMax=-4.04~4.2  SaveName=ScopeData4
  tauz : Scope  NumInputPorts=2
      settings: TimeRange=10  YMin=-1.6e-006~-0.003  YMax=4e-007~0.004  SaveName=ScopeData5
  wires:
  Sum/1 -> Err1/1
  Sum1/1 -> Err2/1
  Sum2/1 -> Err3/1
  Sum3/1 -> Err4/1
  Sum4/1 -> Err5/1
  Sum5/1 -> Err6/1
  GeneralForce5/1 -> Demux/1, "Encoder "/1
  Ref_GeneralForce5/1 -> Demux1/1, "Ref "/1
  Demux/1 -> Sum/1, fx/1
  Demux1/1 -> Sum/2, fx/2
  Demux/2 -> "fy "/1, Sum1/1
  Demux/3 -> fz/1, Sum2/1
  Demux/4 -> Sum3/1, taux/1
  Demux/5 -> tauy/1, Sum4/1
  Demux/6 -> tauz/1, Sum5/1
  Demux1/2 -> "fy "/2, Sum1/2
  Demux1/3 -> fz/2, Sum2/2
  Demux1/4 -> Sum3/2, taux/2
  Demux1/5 -> tauy/2, Sum4/2
  Demux1/6 -> tauz/2, Sum5/2

== system EulerPIDJoint_Tmp/Display/GeneralForceDisplay/Jnt6/Display ==
  GeneralForce6 : Inport
  Ref_GeneralForce6 : Inport  Port=2
  Demux : Demux  Outputs=6
  Demux1 : Demux  Outputs=6
  "Encoder " : ToWorkspace  VariableName=EncGenForceJ6  SampleTime=-1  SaveFormat=Structure
  Err{1..6} (6 alike) : Scope
      Err1 settings: SaveName=ScopeData6
      Err2 settings: SaveName=ScopeData7
      Err3 settings: SaveName=ScopeData8
      Err4 settings: SaveName=ScopeData9
      Err5 settings: TimeRange=3  YMin=-2.5  YMax=1  SaveName=ScopeData10
      Err6 settings: SaveName=ScopeData11
  "Ref " : ToWorkspace  VariableName=RefGenForceJ6  SampleTime=-1  SaveFormat=Structure
  Sum{,1..5} (6 alike) : Sum  Inputs=+|-
  fx : Scope  NumInputPorts=2
      settings: TimeRange=10  YMin=-2.999999999999999e-017~-1  YMax=4e-017~1
  "fy " : Scope  NumInputPorts=2
      settings: YMin=-5~-5  YMax=5~5
  fz : Scope  NumInputPorts=2
      settings: YMin=-5~-5  YMax=5~5  SaveName=ScopeData2
  taux : Scope  NumInputPorts=2
      settings: YMin=-5~-5  YMax=5~5  SaveName=ScopeData3
  tauy : Scope  NumInputPorts=2
      settings: TimeRange=10  YMin=-4.18~4.060000000000001  YMax=-4.04~4.2  SaveName=ScopeData4
  tauz : Scope  NumInputPorts=2
      settings: TimeRange=10  YMin=-1.6e-006~-0.003  YMax=4e-007~0.004  SaveName=ScopeData5
  wires:
  Sum/1 -> Err1/1
  Sum1/1 -> Err2/1
  Sum2/1 -> Err3/1
  Sum3/1 -> Err4/1
  Sum4/1 -> Err5/1
  Sum5/1 -> Err6/1
  GeneralForce6/1 -> Demux/1, "Encoder "/1
  Ref_GeneralForce6/1 -> Demux1/1, "Ref "/1
  Demux/1 -> Sum/1, fx/1
  Demux1/1 -> Sum/2, fx/2
  Demux/2 -> "fy "/1, Sum1/1
  Demux/3 -> fz/1, Sum2/1
  Demux/4 -> Sum3/1, taux/1
  Demux/5 -> tauy/1, Sum4/1
  Demux/6 -> tauz/1, Sum5/1
  Demux1/2 -> "fy "/2, Sum1/2
  Demux1/3 -> fz/2, Sum2/2
  Demux1/4 -> Sum3/2, taux/2
  Demux1/5 -> tauy/2, Sum4/2
  Demux1/6 -> tauz/2, Sum5/2

== system EulerPIDJoint_Tmp/Display/GeneralVelDisplay/Jnt1/Display ==
  GeneralVel1 : Inport
  Ref_GeneralVel1 : Inport  Port=2
  Demux : Demux  Outputs=6
  Demux1 : Demux  Outputs=6
  "Encoder " : ToWorkspace  VariableName=EncGenVelJ1  SampleTime=-1  SaveFormat=Structure
  Err{1..6} (6 alike) : Scope
      Err1 settings: SaveName=ScopeData6
      Err2 settings: SaveName=ScopeData7
      Err3 settings: SaveName=ScopeData8
      Err4 settings: SaveName=ScopeData9
      Err5 settings: TimeRange=3  YMin=-2.5  YMax=1  SaveName=ScopeData10
      Err6 settings: SaveName=ScopeData11
  "Ref " : ToWorkspace  VariableName=RefGenVelJ1  SampleTime=-1  SaveFormat=Structure
  Sum{,1..5} (6 alike) : Sum  Inputs=+|-
  Vx : Scope  NumInputPorts=2
      settings: TimeRange=10  YMin=-2.999999999999999e-017~-1  YMax=4e-017~1
  "Vy " : Scope  NumInputPorts=2
      settings: YMin=-5~-5  YMax=5~5
  Vz : Scope  NumInputPorts=2
      settings: YMin=-5~-5  YMax=5~5  SaveName=ScopeData2
  Wx : Scope  NumInputPorts=2
      settings: YMin=-5~-5  YMax=5~5  SaveName=ScopeData3
  Wy : Scope  NumInputPorts=2
      settings: TimeRange=10  YMin=-4.18~4.060000000000001  YMax=-4.04~4.2  SaveName=ScopeData4
  Wz : Scope  NumInputPorts=2
      settings: TimeRange=10  YMin=-1.6e-006~-0.003  YMax=4e-007~0.004  SaveName=ScopeData5
  wires:
  Sum/1 -> Err1/1
  Sum1/1 -> Err2/1
  Sum2/1 -> Err3/1
  Sum3/1 -> Err4/1
  Sum4/1 -> Err5/1
  Sum5/1 -> Err6/1
  GeneralVel1/1 -> Demux/1, "Encoder "/1
  Ref_GeneralVel1/1 -> Demux1/1, "Ref "/1
  Demux/1 -> Sum/1, Vx/1
  Demux1/1 -> Sum/2, Vx/2
  Demux/2 -> "Vy "/1, Sum1/1
  Demux/3 -> Vz/1, Sum2/1
  Demux/4 -> Sum3/1, Wx/1
  Demux/5 -> Wy/1, Sum4/1
  Demux/6 -> Wz/1, Sum5/1
  Demux1/2 -> "Vy "/2, Sum1/2
  Demux1/3 -> Vz/2, Sum2/2
  Demux1/4 -> Sum3/2, Wx/2
  Demux1/5 -> Wy/2, Sum4/2
  Demux1/6 -> Wz/2, Sum5/2

== system EulerPIDJoint_Tmp/Display/GeneralVelDisplay/Jnt2/Display ==
  GeneralVel2 : Inport
  Ref_GeneralVel2 : Inport  Port=2
  Demux : Demux  Outputs=6
  Demux1 : Demux  Outputs=6
  "Encoder " : ToWorkspace  VariableName=EncGenVelJ2  SampleTime=-1  SaveFormat=Structure
  Err{1..6} (6 alike) : Scope
      Err1 settings: SaveName=ScopeData6
      Err2 settings: SaveName=ScopeData7
      Err3 settings: SaveName=ScopeData8
      Err4 settings: SaveName=ScopeData9
      Err5 settings: TimeRange=3  YMin=-2.5  YMax=1  SaveName=ScopeData10
      Err6 settings: SaveName=ScopeData11
  "Ref " : ToWorkspace  VariableName=RefGenVelJ2  SampleTime=-1  SaveFormat=Structure
  Sum{,1..5} (6 alike) : Sum  Inputs=+|-
  Vx : Scope  NumInputPorts=2
      settings: TimeRange=10  YMin=-2.999999999999999e-017~-1  YMax=4e-017~1
  "Vy " : Scope  NumInputPorts=2
      settings: YMin=-5~-5  YMax=5~5
  Vz : Scope  NumInputPorts=2
      settings: YMin=-5~-5  YMax=5~5  SaveName=ScopeData2
  Wx : Scope  NumInputPorts=2
      settings: YMin=-5~-5  YMax=5~5  SaveName=ScopeData3
  Wy : Scope  NumInputPorts=2
      settings: TimeRange=10  YMin=-4.18~4.060000000000001  YMax=-4.04~4.2  SaveName=ScopeData4
  Wz : Scope  NumInputPorts=2
      settings: TimeRange=10  YMin=-1.6e-006~-0.003  YMax=4e-007~0.004  SaveName=ScopeData5
  wires:
  Demux1/6 -> Sum5/2, Wz/2
  Demux1/5 -> Sum4/2, Wy/2
  Demux1/4 -> Wx/2, Sum3/2
  Demux1/3 -> Sum2/2, Vz/2
  Demux1/2 -> Sum1/2, "Vy "/2
  Demux/6 -> Sum5/1, Wz/1
  Demux/5 -> Sum4/1, Wy/1
  Demux/4 -> Wx/1, Sum3/1
  Demux/3 -> Sum2/1, Vz/1
  Demux/2 -> Sum1/1, "Vy "/1
  Demux1/1 -> Vx/2, Sum/2
  Demux/1 -> Vx/1, Sum/1
  Ref_GeneralVel2/1 -> "Ref "/1, Demux1/1
  GeneralVel2/1 -> "Encoder "/1, Demux/1
  Sum5/1 -> Err6/1
  Sum4/1 -> Err5/1
  Sum3/1 -> Err4/1
  Sum2/1 -> Err3/1
  Sum1/1 -> Err2/1
  Sum/1 -> Err1/1

== system EulerPIDJoint_Tmp/Display/GeneralVelDisplay/Jnt3/Display ==
  GeneralVel3 : Inport
  Ref_GeneralVel3 : Inport  Port=2
  Demux : Demux  Outputs=6
  Demux1 : Demux  Outputs=6
  "Encoder " : ToWorkspace  VariableName=EncGenVelJ3  SampleTime=-1  SaveFormat=Structure
  Err{1..6} (6 alike) : Scope
      Err1 settings: SaveName=ScopeData6
      Err2 settings: SaveName=ScopeData7
      Err3 settings: SaveName=ScopeData8
      Err4 settings: SaveName=ScopeData9
      Err5 settings: TimeRange=3  YMin=-2.5  YMax=1  SaveName=ScopeData10
      Err6 settings: SaveName=ScopeData11
  "Ref " : ToWorkspace  VariableName=RefGenVelJ3  SampleTime=-1  SaveFormat=Structure
  Sum{,1..5} (6 alike) : Sum  Inputs=+|-
  Vx : Scope  NumInputPorts=2
      settings: TimeRange=10  YMin=-2.999999999999999e-017~-1  YMax=4e-017~1
  "Vy " : Scope  NumInputPorts=2
      settings: YMin=-5~-5  YMax=5~5
  Vz : Scope  NumInputPorts=2
      settings: YMin=-5~-5  YMax=5~5  SaveName=ScopeData2
  Wx : Scope  NumInputPorts=2
      settings: YMin=-5~-5  YMax=5~5  SaveName=ScopeData3
  Wy : Scope  NumInputPorts=2
      settings: TimeRange=10  YMin=-4.18~4.060000000000001  YMax=-4.04~4.2  SaveName=ScopeData4
  Wz : Scope  NumInputPorts=2
      settings: TimeRange=10  YMin=-1.6e-006~-0.003  YMax=4e-007~0.004  SaveName=ScopeData5
  wires:
  Sum/1 -> Err1/1
  Sum1/1 -> Err2/1
  Sum2/1 -> Err3/1
  Sum3/1 -> Err4/1
  Sum4/1 -> Err5/1
  Sum5/1 -> Err6/1
  GeneralVel3/1 -> Demux/1, "Encoder "/1
  Ref_GeneralVel3/1 -> Demux1/1, "Ref "/1
  Demux/1 -> Sum/1, Vx/1
  Demux1/1 -> Sum/2, Vx/2
  Demux/2 -> "Vy "/1, Sum1/1
  Demux/3 -> Vz/1, Sum2/1
  Demux/4 -> Sum3/1, Wx/1
  Demux/5 -> Wy/1, Sum4/1
  Demux/6 -> Wz/1, Sum5/1
  Demux1/2 -> "Vy "/2, Sum1/2
  Demux1/3 -> Vz/2, Sum2/2
  Demux1/4 -> Sum3/2, Wx/2
  Demux1/5 -> Wy/2, Sum4/2
  Demux1/6 -> Wz/2, Sum5/2

== system EulerPIDJoint_Tmp/Display/GeneralVelDisplay/Jnt4/Display ==
  GeneralVel4 : Inport
  Ref_GeneralVel4 : Inport  Port=2
  Demux : Demux  Outputs=6
  Demux1 : Demux  Outputs=6
  "Encoder " : ToWorkspace  VariableName=EncGenVelJ4  SampleTime=-1  SaveFormat=Structure
  Err{1..6} (6 alike) : Scope
      Err1 settings: SaveName=ScopeData6
      Err2 settings: SaveName=ScopeData7
      Err3 settings: SaveName=ScopeData8
      Err4 settings: SaveName=ScopeData9
      Err5 settings: TimeRange=3  YMin=-2.5  YMax=1  SaveName=ScopeData10
      Err6 settings: SaveName=ScopeData11
  "Ref " : ToWorkspace  VariableName=RefGenVelJ4  SampleTime=-1  SaveFormat=Structure
  Sum{,1..5} (6 alike) : Sum  Inputs=+|-
  Vx : Scope  NumInputPorts=2
      settings: TimeRange=10  YMin=-2.999999999999999e-017~-1  YMax=4e-017~1
  "Vy " : Scope  NumInputPorts=2
      settings: YMin=-5~-5  YMax=5~5
  Vz : Scope  NumInputPorts=2
      settings: YMin=-5~-5  YMax=5~5  SaveName=ScopeData2
  Wx : Scope  NumInputPorts=2
      settings: YMin=-5~-5  YMax=5~5  SaveName=ScopeData3
  Wy : Scope  NumInputPorts=2
      settings: TimeRange=10  YMin=-4.18~4.060000000000001  YMax=-4.04~4.2  SaveName=ScopeData4
  Wz : Scope  NumInputPorts=2
      settings: TimeRange=10  YMin=-1.6e-006~-0.003  YMax=4e-007~0.004  SaveName=ScopeData5
  wires:
  Demux1/6 -> Sum5/2, Wz/2
  Demux1/5 -> Sum4/2, Wy/2
  Demux1/4 -> Wx/2, Sum3/2
  Demux1/3 -> Sum2/2, Vz/2
  Demux1/2 -> Sum1/2, "Vy "/2
  Demux/6 -> Sum5/1, Wz/1
  Demux/5 -> Sum4/1, Wy/1
  Demux/4 -> Wx/1, Sum3/1
  Demux/3 -> Sum2/1, Vz/1
  Demux/2 -> Sum1/1, "Vy "/1
  Demux1/1 -> Vx/2, Sum/2
  Demux/1 -> Vx/1, Sum/1
  Ref_GeneralVel4/1 -> "Ref "/1, Demux1/1
  GeneralVel4/1 -> "Encoder "/1, Demux/1
  Sum5/1 -> Err6/1
  Sum4/1 -> Err5/1
  Sum3/1 -> Err4/1
  Sum2/1 -> Err3/1
  Sum1/1 -> Err2/1
  Sum/1 -> Err1/1

== system EulerPIDJoint_Tmp/Display/GeneralVelDisplay/Jnt5/Display ==
  GeneralVel5 : Inport
  Ref_GeneralVel5 : Inport  Port=2
  Demux : Demux  Outputs=6
  Demux1 : Demux  Outputs=6
  "Encoder " : ToWorkspace  VariableName=EncGenVelJ5  SampleTime=-1  SaveFormat=Structure
  Err{1..6} (6 alike) : Scope
      Err1 settings: SaveName=ScopeData6
      Err2 settings: SaveName=ScopeData7
      Err3 settings: SaveName=ScopeData8
      Err4 settings: SaveName=ScopeData9
      Err5 settings: TimeRange=3  YMin=-2.5  YMax=1  SaveName=ScopeData10
      Err6 settings: SaveName=ScopeData11
  "Ref " : ToWorkspace  VariableName=RefGenVelJ5  SampleTime=-1  SaveFormat=Structure
  Sum{,1..5} (6 alike) : Sum  Inputs=+|-
  Vx : Scope  NumInputPorts=2
      settings: TimeRange=10  YMin=-2.999999999999999e-017~-1  YMax=4e-017~1
  "Vy " : Scope  NumInputPorts=2
      settings: YMin=-5~-5  YMax=5~5
  Vz : Scope  NumInputPorts=2
      settings: YMin=-5~-5  YMax=5~5  SaveName=ScopeData2
  Wx : Scope  NumInputPorts=2
      settings: YMin=-5~-5  YMax=5~5  SaveName=ScopeData3
  Wy : Scope  NumInputPorts=2
      settings: TimeRange=10  YMin=-4.18~4.060000000000001  YMax=-4.04~4.2  SaveName=ScopeData4
  Wz : Scope  NumInputPorts=2
      settings: TimeRange=10  YMin=-1.6e-006~-0.003  YMax=4e-007~0.004  SaveName=ScopeData5
  wires:
  Sum/1 -> Err1/1
  Sum1/1 -> Err2/1
  Sum2/1 -> Err3/1
  Sum3/1 -> Err4/1
  Sum4/1 -> Err5/1
  Sum5/1 -> Err6/1
  GeneralVel5/1 -> Demux/1, "Encoder "/1
  Ref_GeneralVel5/1 -> Demux1/1, "Ref "/1
  Demux/1 -> Sum/1, Vx/1
  Demux1/1 -> Sum/2, Vx/2
  Demux/2 -> "Vy "/1, Sum1/1
  Demux/3 -> Vz/1, Sum2/1
  Demux/4 -> Sum3/1, Wx/1
  Demux/5 -> Wy/1, Sum4/1
  Demux/6 -> Wz/1, Sum5/1
  Demux1/2 -> "Vy "/2, Sum1/2
  Demux1/3 -> Vz/2, Sum2/2
  Demux1/4 -> Sum3/2, Wx/2
  Demux1/5 -> Wy/2, Sum4/2
  Demux1/6 -> Wz/2, Sum5/2
